simulink model "Task3_Sine_Wave_Adding_Logic"  (R2024b)
settings: Solver=VariableStepAuto  StartTime=0.0  StopTime=10.0  RelTol=1e-3
settings Model: Creator=Ahmad  LastModifiedBy=Ahmad

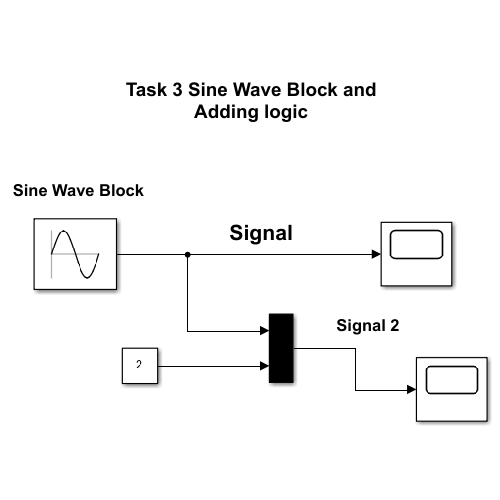
[thumbnail: Simulink's stored preview of the top-level diagram]
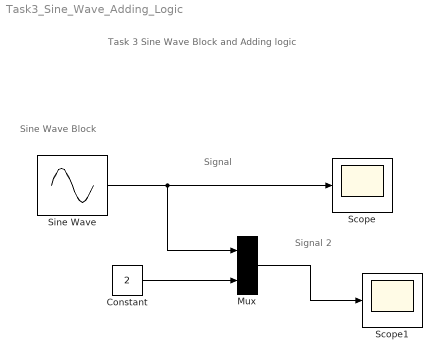
== system Task3_Sine_Wave_Adding_Logic ==
  note: Task 3 Sine Wave Block and Adding logic
  note: Signal 2
  note: Sine Wave Block
  note: Signal
  Constant : Constant  Value=2
  Mux : Mux  Inputs=2
  Scope : Scope
  Scope1 : Scope
  Sine Wave : Sin  Amplitude=5  Frequency=2*pi  SampleTime=0
  wires:
  Sine Wave/1 -> Mux/1, Scope/1
  Constant/1 -> Mux/2
  Mux/1 -> Scope1/1
